simulink model "simulink_control"  (R2024a)
settings: Solver=ode4  StartTime=0.0  StopTime=inf  FixedStep=0.016  RelTol=1e-3
values from neighbouring files (symbols this model uses):
  accelerometer_sensor = wb_robot_get_device('accelerometer')    [simulink_control_app.m]
  alpha_pitch = 0.85    [simulink_control_app.m]
  gps_sensor = wb_robot_get_device('gps')    [simulink_control_app.m]
  gyro_sensor = wb_robot_get_device('gyro')    [simulink_control_app.m]
  inertial_unit = wb_robot_get_device('inertial_unit')    [simulink_control_app.m]
  left_trushter_motor = wb_robot_get_device('left_motor')    [simulink_control_app.m]
  mission_waypoints = [ ... (first row only)    [waypoints.m]
  right_trushter_motor = wb_robot_get_device('right_motor')    [simulink_control_app.m]
  TIME_STEP = 16    [simulink_control_app.m]
libraries: simulink_extras x7, eeGeneralControl x3
settings Model: Creator=Harun  LastModifiedBy=jswku
settings DebuggingCC: UnderSpecifiedDimensionMsg=warning

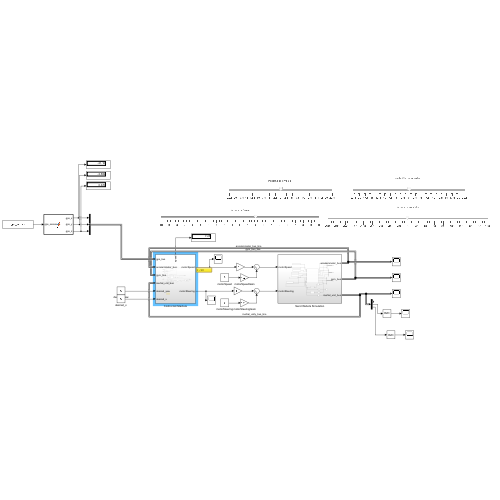
[thumbnail: Simulink's stored preview of the top-level diagram]
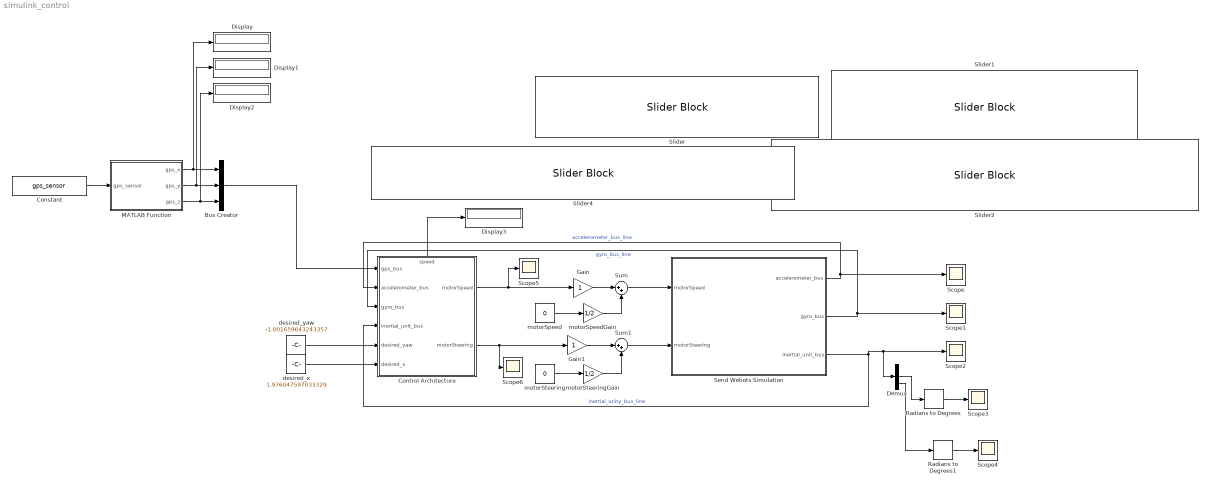
== system simulink_control ==
  Bus Creator : BusCreator  Inputs=3
  Constant : Constant  Value=gps_sensor
  Control Architecture : Subsystem
      settings: PortSchema="{\"entries\":[{\"content\":{\"sides\":[{\"content\":{\"connectorIds\":[\"In1\",\"In2\",\"In3\",\"In4\",\"In5\",\"In6\"]},\"type\":\"ConnectorPlacement.EquallySpacedRectSide\",\"uuid\":\"b8f1fa4d-709a-4c17-bd87-4bca35b482a4\"},{\"content\":{\"connectorIds\":[\"Out1\",\"Out2\"],\"side\":\"RIGHT\"},\"type\":\"ConnectorPlacement.EquallySpacedRectSide\",\"uuid\":\"6380cbab-70d5-44e4-b640-189543dbb2dd\"},{\"content\":{\"connectorIds\":[\"Out3\"],\"side\":\"TOP\"},\"type\":\"ConnectorPlacement.EquallySpacedRectSide\",\"uuid\":\"6fec8609-b346-4b2d-9a85-9302749d2fb3\"}]},\"type\":\"ConnectorPlacement.EquallySpacedConnector\",\"uuid\":\"a3cdcad0-ad7b-441d-8baa-444c58e92ca7\"}],\"packageUris\":[\"http://schema.mathworks.com/mf0/Connector/R2020b\"],\"version\":\"1.0\"}"
  Demux : Demux  Outputs=3
  Display{,1..3} (4 alike) : Display
  Gain : Gain
  Gain1 : Gain
  MATLAB Function : MATLAB Function  TreatAsAtomicUnit=on
  Radians to Degrees : simulink_extras/Transformations/Radians to Degrees
  Radians to Degrees1 : simulink_extras/Transformations/Radians to Degrees
  Scope{,1..6} (7 alike) : Scope
  Send Webots Simulation : Subsystem
  Slider : SliderBlock  ScaleMin=-22.5  ScaleMax=22.5  TickInterval=2.5
  Slider1 : SliderBlock  ScaleMin=-22.5  ScaleMax=22.5  TickInterval=2.5
  Slider2 : SliderBlock  ScaleMin=-180  ScaleMax=180  TickInterval=20
  Slider4 : SliderBlock  ScaleMin=-10  ScaleMax=10
  Sum : Sum  Inputs=|++
  Sum1 : Sum  Inputs=|++
  desired_x : Constant  Value=1.976047597033329
  desired_yaw : Constant  Value=-1.001659643243357
  motorSpeed : Constant  Value=0
  motorSpeedGain : Gain  Gain=1/2
  motorSteering : Constant  Value=0
  motorSteeringGain : Gain  Gain=1/2
  wires:
  motorSteering/1 -> motorSteeringGain/1
  motorSpeed/1 -> motorSpeedGain/1
  Sum/1 -> Send Webots Simulation/1(motorSpeed)
  Control Architecture/1(motorSpeed) -> Scope5/1, Gain/1
  Control Architecture/2(motorSteering) -> Scope6/1, Gain1/1
  Sum1/1 -> Send Webots Simulation/2(motorSteering)
  motorSpeedGain/1 -> Sum/2
  motorSteeringGain/1 -> Sum1/2
  Send Webots Simulation/1(accelerometer_bus) -> Control Architecture/2(accelerometer_bus), Scope/1  "accelerometer_bus_line"
  Send Webots Simulation/2(gyro_bus) -> Control Architecture/3(gyro_bus), Scope1/1  "gyro_bus_line"
  Send Webots Simulation/3(inertial_unit_bus) -> Demux/1, Scope2/1, Control Architecture/4(inertial_unit_bus)  "inertial_unity_bus_line"
  Gain/1 -> Sum/1
  Demux/2 -> Radians to Degrees/1
  Radians to Degrees/1 -> Scope3/1
  Radians to Degrees1/1 -> Scope4/1
  Demux/3 -> Radians to Degrees1/1
  Gain1/1 -> Sum1/1
  desired_x/1 -> Control Architecture/6(desired_x)
  desired_yaw/1 -> Control Architecture/5(desired_yaw)
  Constant/1 -> MATLAB Function/1(gps_sensor)
  MATLAB Function/2(gps_y) -> Display1/1, Bus Creator/2
  MATLAB Function/3(gps_z) -> Display2/1, Bus Creator/3
  MATLAB Function/1(gps_x) -> Display/1, Bus Creator/1
  Bus Creator/1 -> Control Architecture/1(gps_bus)
  Control Architecture/3(speed) -> Display3/1

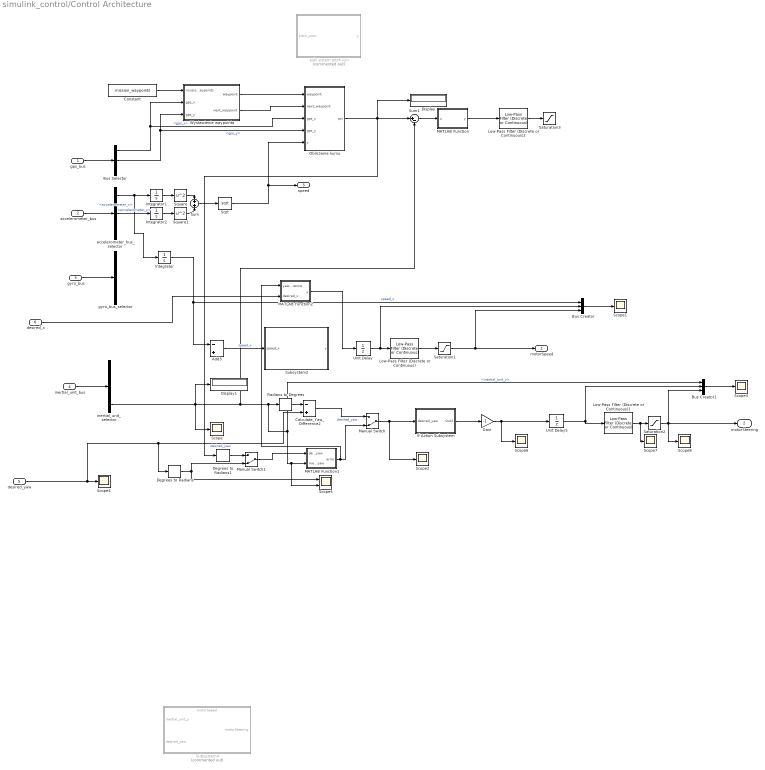
== system simulink_control/Control Architecture ==
  gps_bus : Inport
  accelerometer_bus : Inport  Port=2
  gyro_bus : Inport  Port=3
  inertial_unit_bus : Inport  Port=4
  desired_yaw : Inport  Port=5
  desired_x : Inport  Port=6
  Add3 : Sum  Inputs=-+
  Bus Creator : BusCreator  Inputs=3
  Bus Creator1 : BusCreator  Inputs=3
  Bus Selector : BusSelector  OutputSignals=gps_x,gps_y,gps_z
  Calculate_Yaw_Difference2 : Sum  Inputs=-+
  Constant : Constant  Value=mission_waypoints
  Degrees to Radians : simulink_extras/Transformations/Degrees to Radians
  Degrees to Radians1 : simulink_extras/Transformations/Degrees to Radians
  Display : Display
  Display1 : Display
  Gain : Gain  Gain=-1
  If Action Subsystem : Subsystem  TreatAsAtomicUnit=on
  Integrator : Integrator
  Integrator1 : Integrator
  Integrator2 : Integrator
  Low-Pass Filter (Discrete or Continuous) : eeGeneralControl/Low-Pass Filter (Discrete or Continuous)  K=1  T=0.016  B=inf  A=-inf  init_option=Inherited from block input  x0=0  Ts=-1
  Low-Pass Filter (Discrete or Continuous)1 : eeGeneralControl/Low-Pass Filter (Discrete or Continuous)  K=1  T=0.016  B=inf  A=-inf  init_option=Inherited from block input  x0=0  Ts=-1
  Low-Pass Filter (Discrete or Continuous)2 : eeGeneralControl/Low-Pass Filter (Discrete or Continuous)  K=1  T=0.016  B=inf  A=-inf  init_option=Inherited from block input  x0=0  Ts=-1
  MATLAB Function : MATLAB Function  TreatAsAtomicUnit=on
  MATLAB Function1 : MATLAB Function  TreatAsAtomicUnit=on
  MATLAB Function2 : MATLAB Function  TreatAsAtomicUnit=on
  Manual Switch : ManualSwitch  CurrentSetting=0
  Manual Switch1 : ManualSwitch  CurrentSetting=0
  Obliczenie kursu : MATLAB Function  TreatAsAtomicUnit=on
  Radians to Degrees : simulink_extras/Transformations/Radians to Degrees
  Saturation1 : Saturate  UpperLimit=15  LowerLimit=-15
  Saturation2 : Saturate  UpperLimit=5  LowerLimit=-5
  Saturation3 : Saturate  UpperLimit=15  LowerLimit=-15
  Scope{,1..4,6..8} (8 alike) : Scope
  Scope5 : Scope  NumInputPorts=2
  Sqrt : Sqrt
  Square : Math  Operator=square
  Square1 : Math  Operator=square
  Subsystem2 : Subsystem
  Subsystem4 : Subsystem  Commented=on
      settings: PortSchema="{\"entries\":[{\"content\":{\"sides\":[{\"content\":{\"connectorIds\":[\"In1\",\"In2\"]},\"type\":\"ConnectorPlacement.EquallySpacedRectSide\",\"uuid\":\"8ea77c90-69e3-4b28-847a-36c3733c4ca1\"},{\"content\":{\"connectorIds\":[\"Out1\"],\"side\":\"RIGHT\"},\"type\":\"ConnectorPlacement.EquallySpacedRectSide\",\"uuid\":\"94f1f4b2-c797-44bf-abc2-6d3fe195cf34\"},{\"content\":{\"connectorIds\":[\"In3\"],\"side\":\"TOP\"},\"type\":\"ConnectorPlacement.EquallySpacedRectSide\",\"uuid\":\"06572095-9567-46cb-bcf7-b6a4abacf0e1\"}]},\"type\":\"ConnectorPlacement.EquallySpacedConnector\",\"uuid\":\"9f096835-0cc4-4d1f-8b4a-1f4eeb97a32d\"}],\"packageUris\":[\"http://schema.mathworks.com/mf0/Connector/R2020b\"],\"version\":\"1.0\"}"
  Sum : Sum
  Sum1 : Sum  Inputs=|+-
  Unit Delay : UnitDelay  SampleTime=-1  HasFrameUpgradeWarning=on
  Unit Delay5 : UnitDelay  SampleTime=-1  HasFrameUpgradeWarning=on
  Wystawienie waypointa : MATLAB Function  TreatAsAtomicUnit=on
  accelerometer_bus_selector : BusSelector  OutputSignals=accelerometer_x,accelerometer_y,accelerometer_z
  eski sistem pitch için : Subsystem  Commented=on
  gyro_bus_selector : BusSelector  OutputSignals=gyro_x,gyro_y,gyro_z
  inertial_unit_selector : BusSelector  OutputSignals=inertial_unit_x,inertial_unit_y,inertial_unit_z
  motorSpeed : Outport
  motorSteering : Outport  Port=2
  speed : Outport  Port=3
  wires:
  accelerometer_bus/1 -> accelerometer_bus_selector/1
  gyro_bus/1 -> gyro_bus_selector/1
  inertial_unit_bus/1 -> inertial_unit_selector/1
  Bus Creator/1 -> Scope1/1
  inertial_unit_selector/3 -> Scope/1, Display1/1, Sum1/2, Radians to Degrees/1, Bus Creator1/1, Scope5/2, MATLAB Function1/2(measured_yaw)  "<inertial_unit_z>"
  Saturation1/1 -> motorSpeed/1, Bus Creator/3
  Add3/1 -> Subsystem2/1(speed_x)  "speed_x"
  Integrator/1 -> Add3/1, Bus Creator/1  "speed_x"
  Unit Delay/1 -> Bus Creator/2, Low-Pass Filter (Discrete or Continuous)/1
  Low-Pass Filter (Discrete or Continuous)/1 -> Saturation1/1
  Unit Delay5/1 -> Low-Pass Filter (Discrete or Continuous)1/1, Bus Creator1/2
  Bus Creator1/1 -> Scope3/1
  desired_x/1 -> MATLAB Function2/2(desired_x)
  accelerometer_bus_selector/1 -> Integrator1/1, Integrator/1  "<accelerometer_x>"
  gps_bus/1 -> Bus Selector/1
  Constant/1 -> Wystawienie waypointa/1(mission_waypoints)
  Bus Selector/1 -> Obliczenie kursu/3(gps_x), Wystawienie waypointa/2(gps_x)  "<gps_x>"
  Bus Selector/2 -> Wystawienie waypointa/3(gps_y), Obliczenie kursu/4(gps_y)  "<gps_y>"
  Wystawienie waypointa/1(waypoint) -> Obliczenie kursu/1(waypoint)
  Wystawienie waypointa/2(next_waypoint) -> Obliczenie kursu/2(next_waypoint)
  Square/1 -> Sum/1
  Square1/1 -> Sum/2
  Sum/1 -> Sqrt/1
  Integrator1/1 -> Square/1
  Integrator2/1 -> Square1/1
  Gain/1 -> Scope6/1, Unit Delay5/1
  Obliczenie kursu/1(psi) -> Degrees to Radians1/1, Sum1/1, Display/1
  desired_yaw/1 -> Scope4/1, Calculate_Yaw_Difference2/2, Degrees to Radians/1  "desired_yaw"
  Low-Pass Filter (Discrete or Continuous)2/1 -> Saturation3/1
  Sum1/1 -> MATLAB Function/1(u)
  MATLAB Function/1(y) -> Low-Pass Filter (Discrete or Continuous)2/1
  Saturation2/1 -> Scope8/1, motorSteering/1, Bus Creator1/3
  MATLAB Function1/1(error) -> MATLAB Function2/1(yaw_difference), Manual Switch/2
  Manual Switch/1 -> Scope2/1, If Action Subsystem/1(desired_yaw)
  Radians to Degrees/1 -> Calculate_Yaw_Difference2/1
  Degrees to Radians/1 -> Scope5/1, Manual Switch1/2
  Low-Pass Filter (Discrete or Continuous)1/1 -> Scope7/1, Saturation2/1
  If Action Subsystem/1(Out2) -> Gain/1
  Manual Switch1/1 -> MATLAB Function1/1(desired_yaw)
  Degrees to Radians1/1 -> Manual Switch1/1
  Calculate_Yaw_Difference2/1 -> Manual Switch/1  "desired_yaw"
  MATLAB Function2/1(y) -> Unit Delay/1
  Sqrt/1 -> speed/1, Obliczenie kursu/5(v)
  accelerometer_bus_selector/2 -> Integrator2/1  "<accelerometer_y>"

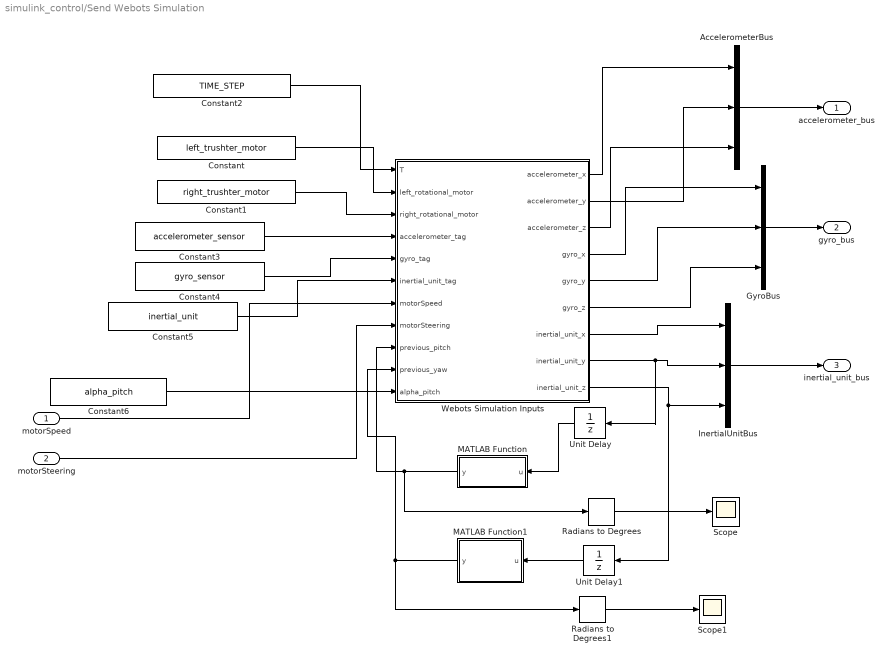
== system simulink_control/Send Webots Simulation ==
  motorSpeed : Inport
  motorSteering : Inport  Port=2
  AccelerometerBus : BusCreator  Inputs=3
  Constant : Constant  Value=left_trushter_motor
  Constant1 : Constant  Value=right_trushter_motor
  Constant2 : Constant  Value=TIME_STEP
  Constant3 : Constant  Value=accelerometer_sensor
  Constant4 : Constant  Value=gyro_sensor
  Constant5 : Constant  Value=inertial_unit
  Constant6 : Constant  Value=alpha_pitch
  GyroBus : BusCreator  Inputs=3
  InertialUnitBus : BusCreator  Inputs=3
  MATLAB Function : MATLAB Function  TreatAsAtomicUnit=on
  MATLAB Function1 : MATLAB Function  TreatAsAtomicUnit=on
  Radians to Degrees : simulink_extras/Transformations/Radians to Degrees
  Radians to Degrees1 : simulink_extras/Transformations/Radians to Degrees
  Scope : Scope
  Scope1 : Scope
  Unit Delay : UnitDelay  SampleTime=-1  HasFrameUpgradeWarning=on
  Unit Delay1 : UnitDelay  SampleTime=-1  HasFrameUpgradeWarning=on
  Webots Simulation Inputs : MATLAB Function  TreatAsAtomicUnit=on
  accelerometer_bus : Outport
  gyro_bus : Outport  Port=2
  inertial_unit_bus : Outport  Port=3
  wires:
  motorSpeed/1 -> Webots Simulation Inputs/7(motorSpeed)
  Constant1/1 -> Webots Simulation Inputs/3(right_rotational_motor)
  Constant2/1 -> Webots Simulation Inputs/1(T)
  Constant/1 -> Webots Simulation Inputs/2(left_rotational_motor)
  Webots Simulation Inputs/2(accelerometer_y) -> AccelerometerBus/2
  Webots Simulation Inputs/1(accelerometer_x) -> AccelerometerBus/1
  Webots Simulation Inputs/3(accelerometer_z) -> AccelerometerBus/3
  AccelerometerBus/1 -> accelerometer_bus/1
  Constant3/1 -> Webots Simulation Inputs/4(accelerometer_tag)
  motorSteering/1 -> Webots Simulation Inputs/8(motorSteering)
  Constant4/1 -> Webots Simulation Inputs/5(gyro_tag)
  Webots Simulation Inputs/6(gyro_z) -> GyroBus/3
  Webots Simulation Inputs/5(gyro_y) -> GyroBus/2
  GyroBus/1 -> gyro_bus/1
  Webots Simulation Inputs/4(gyro_x) -> GyroBus/1
  Webots Simulation Inputs/7(inertial_unit_x) -> InertialUnitBus/1
  Webots Simulation Inputs/8(inertial_unit_y) -> Unit Delay/1, InertialUnitBus/2
  Webots Simulation Inputs/9(inertial_unit_z) -> Unit Delay1/1, InertialUnitBus/3
  InertialUnitBus/1 -> inertial_unit_bus/1
  Constant5/1 -> Webots Simulation Inputs/6(inertial_unit_tag)
  Constant6/1 -> Webots Simulation Inputs/11(alpha_pitch)
  MATLAB Function/1(y) -> Radians to Degrees/1, Webots Simulation Inputs/9(previous_pitch)
  Unit Delay/1 -> MATLAB Function/1(u)
  Radians to Degrees/1 -> Scope/1
  Unit Delay1/1 -> MATLAB Function1/1(u)
  Radians to Degrees1/1 -> Scope1/1
  MATLAB Function1/1(y) -> Radians to Degrees1/1, Webots Simulation Inputs/10(previous_yaw)

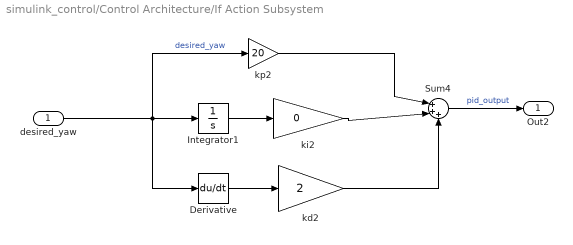
== system simulink_control/Control Architecture/If Action Subsystem ==
  desired_yaw : Inport
  Derivative : Derivative
  Integrator1 : Integrator
  Sum4 : Sum  Inputs=|+++
  kd2 : Gain  Gain=2
  ki2 : Gain  Gain=0
  kp2 : Gain  Gain=20
  Out2 : Outport
  wires:
  Sum4/1 -> Out2/1  "pid_output"
  kp2/1 -> Sum4/1
  ki2/1 -> Sum4/2
  Integrator1/1 -> ki2/1
  desired_yaw/1 -> Derivative/1, kp2/1, Integrator1/1  "desired_yaw"
  kd2/1 -> Sum4/3
  Derivative/1 -> kd2/1

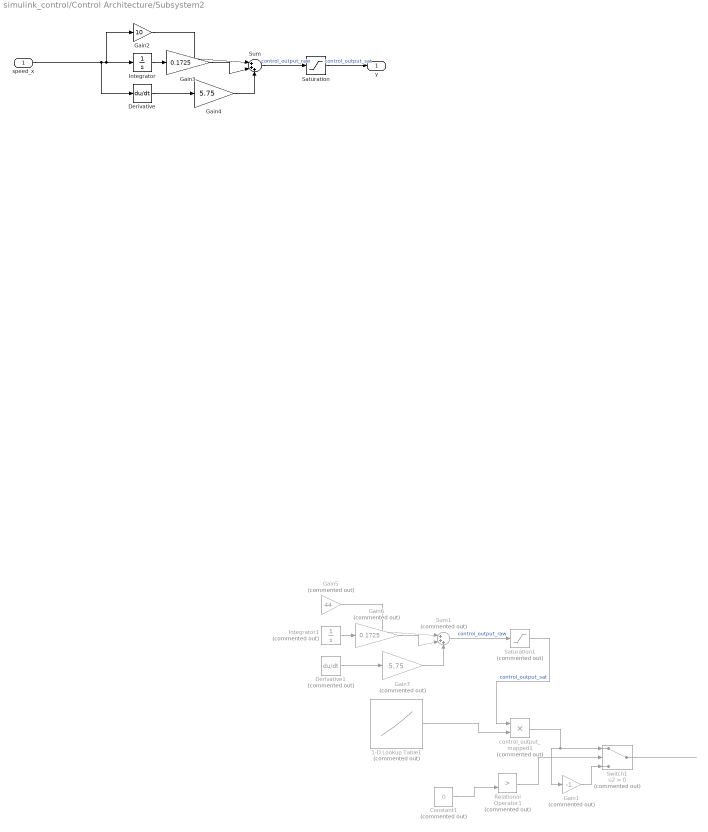
== system simulink_control/Control Architecture/Subsystem2 ==
  speed_x : Inport
  1-D Lookup Table1 : Lookup_n-D  Commented=on  NumberOfTableDimensions=1  BreakpointsForDimension1=|  Table=|  InternalRulePriority=Speed  RndMeth=Simplest
      BreakpointsForDimension1=|
      | [
      | -25.0
      |    -22.5
      |    -20.0
      |    -17.5
      |    -15.0
      |    -12.5
      |    -10.0
      |     -7.5
      |     -5.0
      |     -2.5
      |      0.0
      |      2.5
      |      5.0
      |      7.5
      |     10.0
      |     12.5
      |     15.0
      |     17.5
      |     20.0
      |     22.5
      |     25.0
      | ];
      Table=|
      | [-0.50
      |    -0.45
      |    -0.40
      |    -0.35
      |    -0.30
      |    -0.25
      |    -0.20
      |    -0.15
      |    -0.10
      |    -0.05
      |     0.00
      |     0.05
      |     0.10
      |     0.15
      |     0.20
      |     0.25
      |     0.30
      |     0.35
      |     0.40
      |     0.45
      |     0.50
      | ];
  Constant1 : Constant  Commented=on  Value=0
  Derivative : Derivative  CoefficientInTFapproximation=0.016
  Derivative1 : Derivative  Commented=on  CoefficientInTFapproximation=0.016
  Gain1 : Gain  Commented=on  Gain=-1
  Gain2 : Gain  Gain=10
  Gain3 : Gain  Gain=0.1725
  Gain4 : Gain  Gain=5.75
  Gain5 : Gain  Commented=on  Gain=44
  Gain6 : Gain  Commented=on  Gain=0.1725
  Gain7 : Gain  Commented=on  Gain=5.75
  Integrator : Integrator
  Integrator1 : Integrator  Commented=on
  Relational Operator1 : RelationalOperator  Commented=on  Operator=>  OutDataTypeStr=boolean  RndMeth=Simplest  InputSameDT=off
  Saturation : Saturate  UpperLimit=250  LowerLimit=-250
  Saturation1 : Saturate  Commented=on  UpperLimit=250  LowerLimit=-250
  Sum : Sum  Inputs=|+++
  Sum1 : Sum  Commented=on  Inputs=|+++
  Switch1 : Switch  Commented=on  Criteria=u2 > Threshold  SaturateOnIntegerOverflow=off  InputSameDT=off
  control_output_mapped1 : Product  Commented=on
  y : Outport
  wires:
  Integrator/1 -> Gain3/1
  Gain3/1 -> Sum/2
  Gain2/1 -> Sum/1
  Sum/1 -> Saturation/1  "control_output_raw"
  Derivative/1 -> Gain4/1
  Gain4/1 -> Sum/3
  speed_x/1 -> Derivative/1, Gain2/1, Integrator/1
  ? -> 1-D Lookup Table1/1, Relational Operator1/1, Derivative1/1, Gain5/1, Integrator1/1
  Switch1/1 -> ?
  Relational Operator1/1 -> Switch1/2
  Gain7/1 -> Sum1/3
  Derivative1/1 -> Gain7/1
  Gain1/1 -> Switch1/3
  Gain5/1 -> Sum1/1
  control_output_mapped1/1 -> Gain1/1, Switch1/1
  Sum1/1 -> Saturation1/1  "control_output_raw"
  Constant1/1 -> Relational Operator1/2
  Saturation1/1 -> control_output_mapped1/1  "control_output_sat"
  Integrator1/1 -> Gain6/1
  1-D Lookup Table1/1 -> control_output_mapped1/2
  Gain6/1 -> Sum1/2
  Saturation/1 -> y/1  "control_output_sat"

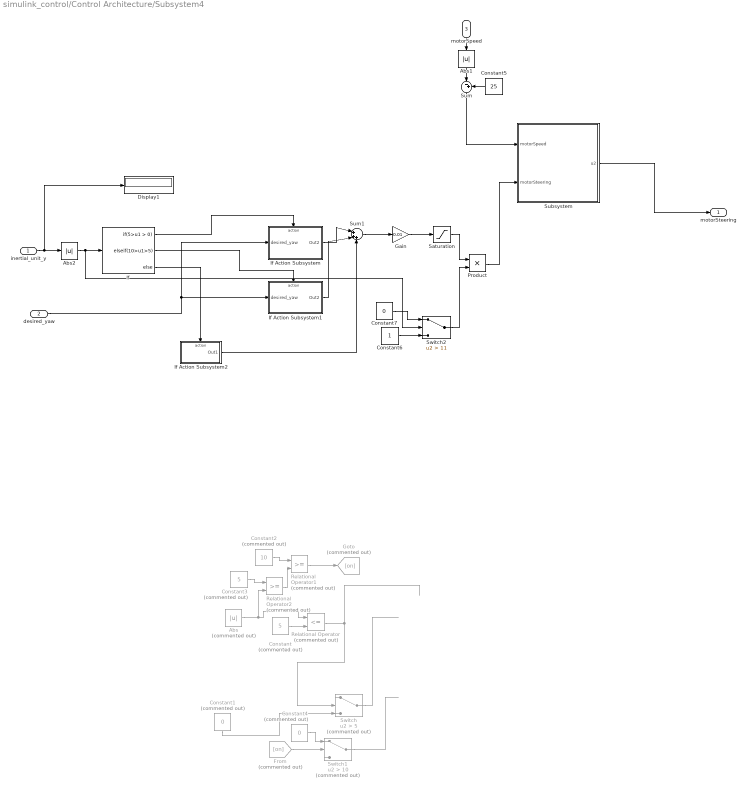
== system simulink_control/Control Architecture/Subsystem4 ==
  inertial_unit_y : Inport
  desired_yaw : Inport  Port=2
  motorSpeed : Inport  Port=3
  Abs : Abs  Commented=on  SaturateOnIntegerOverflow=off
  Abs1 : Abs  SaturateOnIntegerOverflow=off
  Abs2 : Abs  SaturateOnIntegerOverflow=off
  Constant : Constant  Commented=on  Value=5
  Constant1 : Constant  Commented=on  Value=0
  Constant2 : Constant  Commented=on  Value=10
  Constant3 : Constant  Commented=on  Value=5
  Constant4 : Constant  Commented=on  Value=0
  Constant5 : Constant  Value=25
  Constant6 : Constant
  Constant7 : Constant  Value=0
  Display1 : Display
  From : From  Commented=on  GotoTag=on
  Gain : Gain  Gain=0.01
  Goto : Goto  Commented=on  GotoTag=on
  If : If  IfExpression=5>u1 > 0  ElseIfExpressions=10>u1>5
  If Action Subsystem : Subsystem  TreatAsAtomicUnit=on
  If Action Subsystem1 : Subsystem  TreatAsAtomicUnit=on
  If Action Subsystem2 : Subsystem  TreatAsAtomicUnit=on
  Product : Product
  Relational Operator : RelationalOperator  Commented=on  Operator=<=  OutDataTypeStr=boolean  RndMeth=Simplest  InputSameDT=off
  Relational Operator1 : RelationalOperator  Commented=on  OutDataTypeStr=boolean  RndMeth=Simplest  InputSameDT=off
  Relational Operator2 : RelationalOperator  Commented=on  OutDataTypeStr=boolean  RndMeth=Simplest  InputSameDT=off
  Saturation : Saturate  UpperLimit=1000  LowerLimit=-1000
  Subsystem : Subsystem
  Sum : Sum  Inputs=|-+
  Sum1 : Sum  Inputs=|+++
  Switch : Switch  Commented=on  Criteria=u2 > Threshold  Threshold=5  SaturateOnIntegerOverflow=off  InputSameDT=off
  Switch1 : Switch  Commented=on  Criteria=u2 > Threshold  Threshold=10  SaturateOnIntegerOverflow=off  InputSameDT=off
  Switch2 : Switch  Criteria=u2 > Threshold  Threshold=11  SaturateOnIntegerOverflow=off  InputSameDT=off
  motorSteering : Outport
  wires:
  motorSpeed/1 -> Abs1/1
  Abs1/1 -> Sum/1
  Constant5/1 -> Sum/2
  Constant1/1 -> Switch/3
  From/1 -> Switch1/2
  Constant4/1 -> Switch1/1
  Switch1/1 -> ?
  Constant/1 -> Relational Operator/2
  Relational Operator1/1 -> Goto/1
  Constant3/1 -> Relational Operator2/1
  Abs/1 -> Relational Operator2/2, Relational Operator/1
  ? -> Switch1/3, Switch/1
  Constant2/1 -> Relational Operator1/1
  Switch/1 -> ?
  Relational Operator2/1 -> Relational Operator1/2
  Relational Operator/1 -> Switch/2
  inertial_unit_y/1 -> Display1/1, Abs2/1
  If/3 -> If Action Subsystem2/Action
  Abs2/1 -> Switch2/2, If/1
  If/1 -> If Action Subsystem/Action
  If Action Subsystem1/1(Out2) -> Sum1/2
  If Action Subsystem/1(Out2) -> Sum1/1
  If/2 -> If Action Subsystem1/Action
  Sum1/1 -> Gain/1
  Gain/1 -> Saturation/1
  Sum/1 -> Subsystem/1(motorSpeed)
  Saturation/1 -> Product/1
  Constant6/1 -> Switch2/3
  Constant7/1 -> Switch2/1
  Switch2/1 -> Product/2
  Product/1 -> Subsystem/2(motorSteering)
  If Action Subsystem2/1(Out1) -> Sum1/3
  desired_yaw/1 -> If Action Subsystem/1(desired_yaw), If Action Subsystem1/1(desired_yaw)
  Subsystem/1(u2) -> motorSteering/1

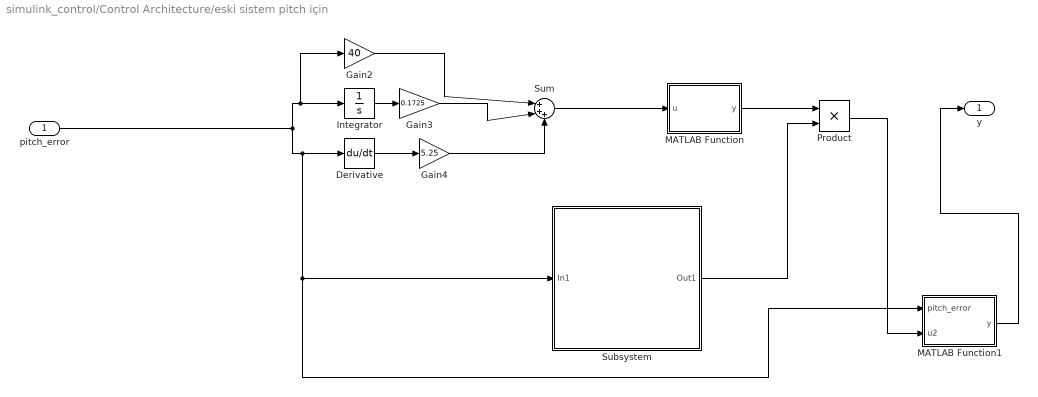
== system simulink_control/Control Architecture/eski sistem pitch için ==
  pitch_error : Inport
  Derivative : Derivative  CoefficientInTFapproximation=0.016
  Gain2 : Gain  Gain=40
  Gain3 : Gain  Gain=0.1725
  Gain4 : Gain  Gain=5.25
  Integrator : Integrator
  MATLAB Function : MATLAB Function  TreatAsAtomicUnit=on
  MATLAB Function1 : MATLAB Function  TreatAsAtomicUnit=on
  Product : Product
  Subsystem : Subsystem
  Sum : Sum  Inputs=|+++
  y : Outport
  wires:
  MATLAB Function1/1(y) -> y/1
  Product/1 -> MATLAB Function1/2(u2)
  MATLAB Function/1(y) -> Product/1
  Sum/1 -> MATLAB Function/1(u)
  Subsystem/1(Out1) -> Product/2
  pitch_error/1 -> Integrator/1, Gain2/1, Derivative/1, MATLAB Function1/1(pitch_error), Subsystem/1(In1)
  Gain4/1 -> Sum/3
  Gain2/1 -> Sum/1
  Gain3/1 -> Sum/2
  Integrator/1 -> Gain3/1
  Derivative/1 -> Gain4/1

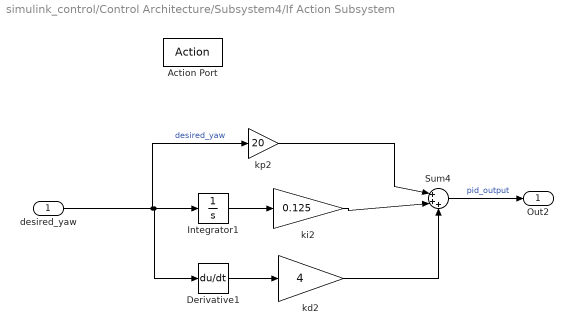
== system simulink_control/Control Architecture/Subsystem4/If Action Subsystem ==
  desired_yaw : Inport
  Action Port : ActionPort
  Derivative1 : Derivative  CoefficientInTFapproximation=0.016
  Integrator1 : Integrator
  Sum4 : Sum  Inputs=|+++
  kd2 : Gain  Gain=4
  ki2 : Gain  Gain=0.125
  kp2 : Gain  Gain=20
  Out2 : Outport
  wires:
  Derivative1/1 -> kd2/1
  Sum4/1 -> Out2/1  "pid_output"
  kp2/1 -> Sum4/1
  ki2/1 -> Sum4/2
  Integrator1/1 -> ki2/1
  desired_yaw/1 -> kp2/1, Derivative1/1, Integrator1/1  "desired_yaw"
  kd2/1 -> Sum4/3

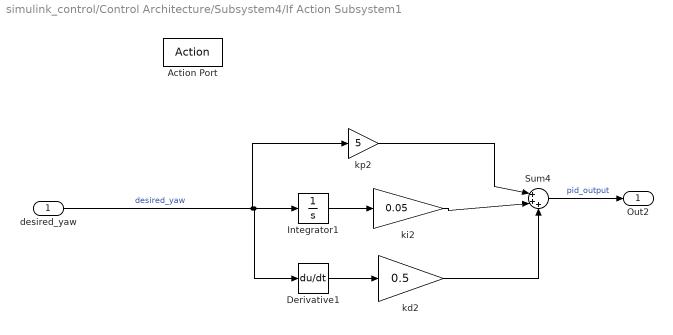
== system simulink_control/Control Architecture/Subsystem4/If Action Subsystem1 ==
  desired_yaw : Inport
  Action Port : ActionPort
  Derivative1 : Derivative  CoefficientInTFapproximation=0.016
  Integrator1 : Integrator
  Sum4 : Sum  Inputs=|+++
  kd2 : Gain  Gain=0.5
  ki2 : Gain  Gain=0.05
  kp2 : Gain  Gain=5
  Out2 : Outport
  wires:
  Derivative1/1 -> kd2/1
  Sum4/1 -> Out2/1  "pid_output"
  kp2/1 -> Sum4/1
  ki2/1 -> Sum4/2
  Integrator1/1 -> ki2/1
  desired_yaw/1 -> kp2/1, Derivative1/1, Integrator1/1  "desired_yaw"
  kd2/1 -> Sum4/3

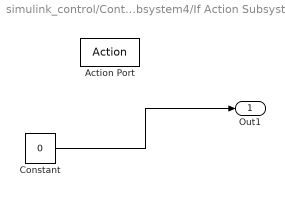
== system simulink_control/Control Architecture/Subsystem4/If Action Subsystem2 ==
  Action Port : ActionPort
  Constant : Constant  Value=0
  Out1 : Outport
  wires:
  Constant/1 -> Out1/1

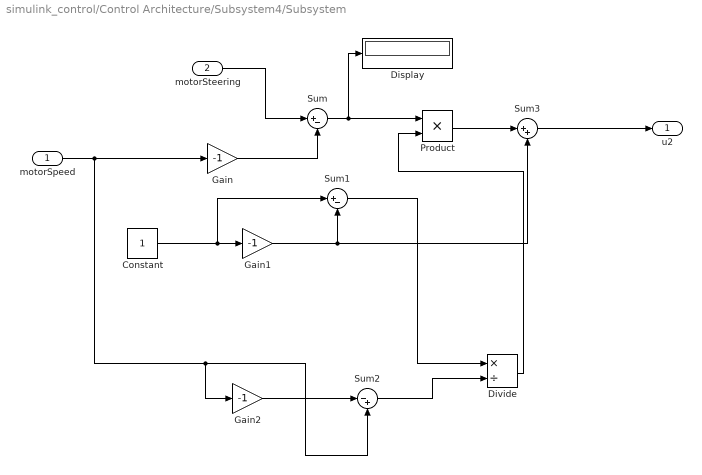
== system simulink_control/Control Architecture/Subsystem4/Subsystem ==
  motorSpeed : Inport
  motorSteering : Inport  Port=2
  Constant : Constant
  Display : Display
  Divide : Product  Inputs=*/
  Gain : Gain  Gain=-1
  Gain1 : Gain  Gain=-1
  Gain2 : Gain  Gain=-1
  Product : Product
  Sum : Sum  Inputs=|+-
  Sum1 : Sum  Inputs=|+-
  Sum2 : Sum  Inputs=|-+
  Sum3 : Sum  Inputs=|++
  u2 : Outport
  wires:
  Sum3/1 -> u2/1
  Product/1 -> Sum3/1
  Divide/1 -> Product/2
  Sum1/1 -> Divide/1
  Sum2/1 -> Divide/2
  Gain2/1 -> Sum2/1
  motorSpeed/1 -> Gain2/1, Sum2/2, Gain/1
  Constant/1 -> Gain1/1, Sum1/1
  Gain1/1 -> Sum1/2, Sum3/2
  Sum/1 -> Display/1, Product/1
  Gain/1 -> Sum/2
  motorSteering/1 -> Sum/1

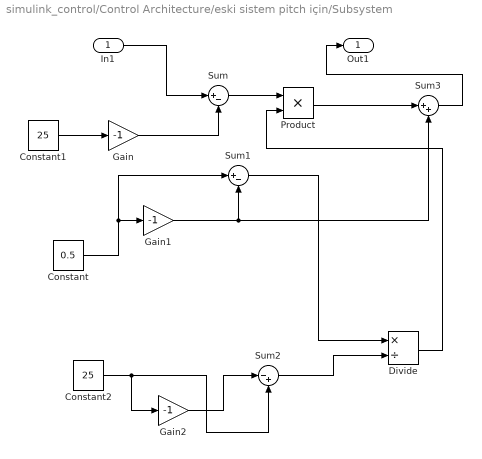
== system simulink_control/Control Architecture/eski sistem pitch için/Subsystem ==
  In1 : Inport
  Constant : Constant  Value=0.5
  Constant1 : Constant  Value=25
  Constant2 : Constant  Value=25
  Divide : Product  Inputs=*/
  Gain : Gain  Gain=-1
  Gain1 : Gain  Gain=-1
  Gain2 : Gain  Gain=-1
  Product : Product
  Sum : Sum  Inputs=|+-
  Sum1 : Sum  Inputs=|+-
  Sum2 : Sum  Inputs=|-+
  Sum3 : Sum  Inputs=|++
  Out1 : Outport
  wires:
  Sum3/1 -> Out1/1
  Product/1 -> Sum3/1
  Divide/1 -> Product/2
  Sum1/1 -> Divide/1
  Sum2/1 -> Divide/2
  Gain2/1 -> Sum2/1
  Constant2/1 -> Gain2/1, Sum2/2
  Constant/1 -> Gain1/1, Sum1/1
  Gain1/1 -> Sum1/2, Sum3/2
  Sum/1 -> Product/1
  Gain/1 -> Sum/2
  Constant1/1 -> Gain/1
  In1/1 -> Sum/1

== matlab function simulink_control/Control Architecture/MATLAB Function ==
  data: u input; y output
function y = fcn(u)

y = u;

== matlab function simulink_control/Control Architecture/MATLAB Function1 ==
  data: desired_yaw input; error output; measured_yaw input
function error = fcn(desired_yaw,measured_yaw)
error = atan2(sin(desired_yaw-measured_yaw),cos(desired_yaw-measured_yaw));

end

== matlab function simulink_control/Control Architecture/MATLAB Function2 ==
  data: yaw_difference input; y output; desired_x input
function y = fcn(yaw_difference, desired_x)

if yaw_difference < 0.01 
    y=desired_x;

elseif yaw_difference > -0.01

    y=desired_x ;
else
    y=desired_x*0.5;
end
end

== matlab function simulink_control/Send Webots Simulation/MATLAB Function1 ==
  data: u input; y output
function y = fcn(u)

y = u;

== matlab function simulink_control/Control Architecture/eski sistem pitch için/MATLAB Function ==
  data: u input; y output
function y = fcn(u)



y = max(-250,min(250,u));
end

== matlab function simulink_control/Control Architecture/eski sistem pitch için/MATLAB Function1 ==
  data: pitch_error input; y output; u2 input
function y = fcn(pitch_error,u2)
if(pitch_error<0)
    y=-u2
else
    y=u2
end

== matlab function simulink_control/MATLAB Function ==
  data: gps_sensor input; gps_x output; gps_y output; gps_z output
function [gps_x, gps_y, gps_z] = fcn(gps_sensor)

coder.extrinsic('wb_gps_get_values');


gps_x = 0;
gps_y = 0;
gps_z = 0;

position=wb_gps_get_values(gps_sensor);

gps_x=position(1);
gps_y=position(2);
gps_z=position(3);

== matlab function simulink_control/Send Webots Simulation/Webots Simulation Inputs ==
  data: T input; left_rotational_motor input; right_rotational_motor input; accelerometer_tag input; gyro_tag input; inertial_unit_tag input; motorSpeed input; accelerometer_x output; accelerometer_y output; accelerometer_z output; motorSteering input; gyro_x output; gyro_y output; gyro_z output; inertial_unit_x output; inertial_unit_y output; inertial_unit_z output; previous_pitch input; previous_yaw input; alpha_pitch input
function [accelerometer_x,accelerometer_y,accelerometer_z,gyro_x,gyro_y,gyro_z,inertial_unit_x,inertial_unit_y,inertial_unit_z] = simulation(T,left_rotational_motor,right_rotational_motor,accelerometer_tag,gyro_tag,inertial_unit_tag ...
    ,motorSpeed,motorSteering,previous_pitch,previous_yaw,alpha_pitch)

accelerometer_x = 0.0;
accelerometer_y = 0.0;
accelerometer_z = 0.0;

gyro_x=0.0;
gyro_y=0.0;
gyro_z=0.0;

wb_robot_step(T)
wb_motor_set_position(left_rotational_motor, Inf);
wb_motor_set_position(right_rotational_motor, Inf);
wb_motor_set_velocity(right_rotational_motor, motorSpeed-motorSteering);
wb_motor_set_velocity(left_rotational_motor, motorSpeed+motorSteering);

%period = wb_accelerometer_get_sampling_period(accelerometer_tag)
accelerometer_values = zeros(1, 3); 
accelerometer_values = wb_accelerometer_get_values(accelerometer_tag);
accelerometer_x = accelerometer_values(1);
accelerometer_y = accelerometer_values(2);
accelerometer_z = accelerometer_values(3);



gyro_values = zeros(1, 3); 
gyro_values = wb_gyro_get_values(gyro_tag);

gyro_x = gyro_values(1);
gyro_y = gyro_values(2);
gyro_z = gyro_values(3);


inertial_unit_values = zeros(1, 3); 
inertial_unit_values = wb_inertial_unit_get_roll_pitch_yaw(inertial_unit_tag);



inertial_unit_x = inertial_unit_values(1);
inertial_unit_y = inertial_unit_values(2);
inertial_unit_z = inertial_unit_values(3);

interial_unit_y=alpha_pitch*inertial_unit_y+(1-alpha_pitch)*previous_pitch;

inertial_unit_z=alpha_pitch*inertial_unit_z+(1-alpha_pitch)*previous_yaw;


end

== matlab function simulink_control/Control Architecture/Wystawienie waypointa ==
  data: mission_waypoints input; waypoint output; gps_x input; gps_y input; next_waypoint output
function [waypoint, next_waypoint] = fcn(mission_waypoints, gps_x, gps_y)

persistent index
if isempty(index)
    index = 1;
end

N = size(mission_waypoints,1);

% zabezpieczenie gdy koniec trasy
if index >= N
    waypoint = mission_waypoints(N,:);
    next_waypoint = mission_waypoints(N,:);   % brak następnego
    return
end

% aktualny waypoint
waypoint = mission_waypoints(index,:);
next_waypoint = mission_waypoints(index+1,:);

ex = waypoint(1) - gps_x;
ey = waypoint(2) - gps_y;

distance = sqrt(ex^2 + ey^2);

if distance < 1
    index = index + 1;
end

end

== matlab function simulink_control/Control Architecture/Obliczenie kursu ==
  data: waypoint input; next_waypoint input; psi output; gps_x input; gps_y input; v input
function psi = fcn(waypoint,next_waypoint,gps_x, gps_y,v)

path_angle=atan2(waypoint(2)-next_waypoint(2),waypoint(1) -next_waypoint(1));

e=-((gps_x-waypoint(1))*sin(path_angle)+(gps_y-waypoint(2)) * cos(path_angle));

delta = 4+2*v;

psi=path_angle+atan(-e/delta);

== matlab function simulink_control/Send Webots Simulation/MATLAB Function ==
  data: u input; y output
function y = fcn(u)

y = u;
